simulink model "two_phase_main_loop"  (R2025b)
settings: Solver=daessc  StartTime=0  StopTime=50000
undefined symbols (not defined in the file): cfg, u_cmd
libraries: fl_lib x38, nesl_utility x26, SimscapeFluids_lib x11, slpidlib x2
(part 2 of 2)

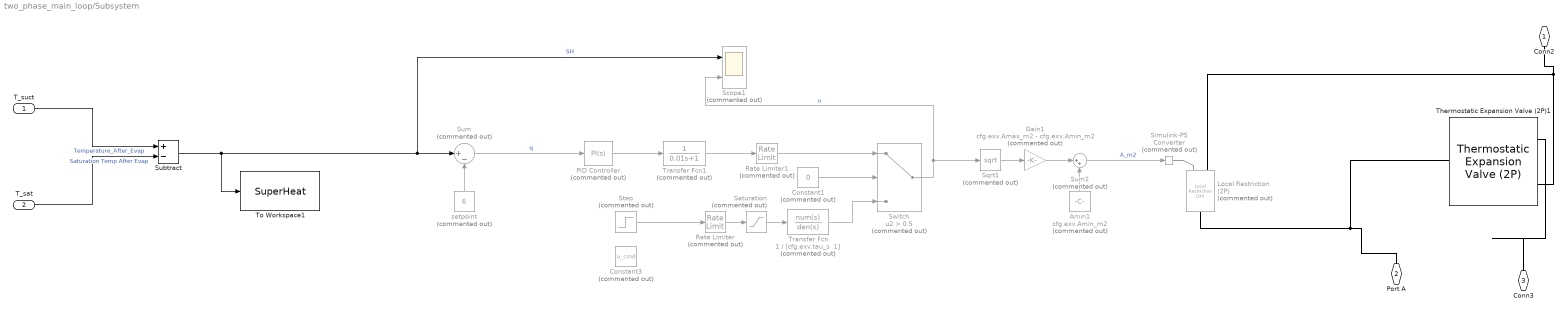
== system two_phase_main_loop/Subsystem ==
  T_suct : Inport
  T_sat : Inport  Port=2
  Amin1 : Constant  Commented=on  Value=cfg.exv.Amin_m2
  Constant1 : Constant  Commented=on  Value=0
  Constant3 : Constant  Commented=on  Value=u_cmd
  Gain1 : Gain  Commented=on  Gain=cfg.exv.Amax_m2 - cfg.exv.Amin_m2
  Local Restriction (2P) : fl_lib/Two-Phase Fluid/Elements/Local Restriction (2P)  Commented=on  restriction_type=foundation.enum.restriction_type.variable  restriction_area=1e-3 m^2  min_area="cfg.exv.Amin_m2  m^2"  max_area="cfg.exv.Amax_m2  m^2"  pressure_loss_model=foundation.enum.RestrictionPressureLossModel.Bernoulli  area=pi*0.02^2/4 m^2  Cd=0.64  B_lam=0.999
      settings: InternalSimscapePortConfiguration="{\"Bottom\":[],\"Left\":[{\"id\":\"A\",\"label\":\"A\",\"type\":\"foundation.two_phase_fluid.two_phase_fluid\"},{\"id\":\"area_in\",\"label\":\"AR\",\"type\":\"input\"}],\"Right\":[{\"id\":\"B\",\"label\":\"B\",\"type\":\"foundation.two_phase_fluid.two_phase_fluid\"}],\"Top\":[]}"
  PID Controller : slpidlib/PID Controller  Commented=on  Controller=PI  Form=Parallel  TimeDomain=Continuous-time  UseExternalTs=off  SampleTime=-1  IntegratorMethod=Forward Euler  FilterMethod=Forward Euler  ControllerParametersSource=internal  P=-0.05  I=- 0.001  UseKiTs=off  D=0  UseExternalDerivativeSource=off  N=100  UseFilter=on  TunerSelectOption=Transfer Function Based (PID Tuner App)  InitialConditionSource=internal  InitialConditionForIntegrator=0  InitialConditionForFilter=0  DifferentiatorICPrevScaledInput=0  ExternalReset=none  TrackingMode=off  Kt=1  LimitOutput=on  SatLimitsSource=internal  UpperSaturationLimit=1  LowerSaturationLimit=0  LinearizeAsGain=on  AntiWindupMode=clamping  Kb=1  LimitIntegrator=on  UpperIntegratorSaturationLimit=1  LowerIntegratorSaturationLimit=0  POutMin=[]  POutMax=[]  IOutMin=[]  IOutMax=[]  DOutMin=[]  DOutMax=[]  NOutMin=[]  NOutMax=[]  SumOutMin=[]  SumOutMax=[]  SaturationOutMin=[]  SaturationOutMax=[]  PParamMin=[]  PParamMax=[]  IParamMin=[]  IParamMax=[]  DParamMin=[]  DParamMax=[]  NParamMin=[]  NParamMax=[]  KbParamMin=[]  KbParamMax=[]  KtParamMin=[]  KtParamMax=[]  KbOutMin=[]  KbOutMax=[]  KtOutMin=[]  KtOutMax=[]  IntegratorOutMin=[]  IntegratorOutMax=[]  FilterOutMin=[]  FilterOutMax=[]  SumI1OutMin=[]  SumI1OutMax=[]  SumI2OutMin=[]  SumI2OutMax=[]  SumI3OutMin=[]  SumI3OutMax=[]  SumI4OutMin=[]  SumI4OutMax=[]  SumDOutMin=[]  SumDOutMax=[]  DifferentiatorOutMin=[]  DifferentiatorOutMax=[]  FilterDiffOutCoefMin=[]  FilterDiffOutCoefMax=[]  ReciprocalOutMin=[]  ReciprocalOutMax=[]  SumDenOutMin=[]  SumDenOutMax=[]  SumNumOutMin=[]  SumNumOutMax=[]  DivideOutMin=[]  DivideOutMax=[]  UdiffTsProdOutMin=[]  UdiffTsProdOutMax=[]  NTsProdOutMin=[]  NTsProdOutMax=[]  UintegralTsProdOutMin=[]  UintegralTsProdOutMax=[]  UngainTsProdOutMin=[]  UngainTsProdOutMax=[]  ClampingZeroOutDataTypeStr=Inherit: Inherit via back propagation  ClampingZeroOutMin=[]  ClampingZeroOutMax=[]  FilterDenConstantOutDataTypeStr=Inherit: Inherit via back propagation  FilterDenConstantOutMin=[]  FilterDenConstantOutMax=[]  PCopyOutDataTypeStr=Inherit: Inherit via back propagation  PCopyOutMin=[]  PCopyOutMax=[]  NCopyOutDataTypeStr=Inherit: Inherit via back propagation  NCopyOutMin=[]  NCopyOutMax=[]  IntegratorContinuousStateAttributes=''  IntegratorStateMustResolveToSignalObject=off  IntegratorRTWStateStorageClass=Auto  FilterContinuousStateAttributes=''  FilterStateMustResolveToSignalObject=off  FilterRTWStateStorageClass=Auto  ParallelPVariant=InternalParameters  IdealPVariant=Disabled  IVariant=InternalParameters  DVariant=Disabled  IntegratorVariant=Continuous  SatVariant=Enabled  AWVariant=ContClampingParallel  PCopyVariant=Disabled  TRVariant=Disabled  FdbkBlocksVariant=Forward  IdealPFdbkVariant=Disabled  SatFdbkVariant=Disabled  DerivativeFilterVariant=Disabled  NVariant=Disabled  NCopyVariant=Disabled_SignalSpec  FilterICVariant=Disabled  IntegratorICVariant=InternalICs  ExternalResetVariant=Disabled  TRSumVariant=Passthrough  SumFdbkVariant=Disabled  SumVariant=Sum_PI  TsampFilterVariant=InternalTs  TsampNgainVariant=Passthrough  TsampIntegralVariant=Disabled_SignalSpec  ExternalSaturationOutDataTypeStr=Inherit: Same as second input  DerivativeSourceVariant=Disabled  PreIntVariant=InternalPreInt
  Rate Limiter : RateLimiter  Commented=on  RisingSlewLimit=0.001  FallingSlewLimit=-0.001  SampleTimeMode=inherited  LinearizeAsGain=off
  Rate Limiter1 : RateLimiter  Commented=on  RisingSlewLimit=100  FallingSlewLimit=- 100  SampleTimeMode=inherited  LinearizeAsGain=off
  Saturation : Saturate  Commented=on  UpperLimit=cfg.exv.u_max  LowerLimit=0
  Scope1 : Scope  Commented=on  NumInputPorts=2
      settings: ActiveDisplayYMinimum=-231.24035158922058  ActiveDisplayYMaximum=311.50161349127353  DataLoggingVariableName=ScopeData3
  Simulink-PS Converter : nesl_utility/Simulink-PS Converter  Commented=on  PhysicalDomain=network_engine_domain  SubClassName=ps_input  LeftPortType=input  RightPortType=output  PseudoPeriodic=off  Frequencies=[]  NoiseDistribution=none  NoiseParameters=[]  Unit=m^2  AffineConversion=off  FilteringAndDerivatives=provide  SimscapeFilterOrder=1  InputFilterTimeConstant=0.001  UdotUserProvided=0
  Sqrt1 : Sqrt  Commented=on
  Step : Step  Commented=on  Time=600  Before=0.004  After=0.015  SampleTime=0
  Subtract : Sum  Inputs=+-
  Sum : Sum  Commented=on  Inputs=|+-
  Sum2 : Sum  Commented=on  Inputs=|++
  Switch : Switch  Commented=on  Criteria=u2 > Threshold  Threshold=0.5  SaturateOnIntegerOverflow=off  InputSameDT=off
  Thermostatic Expansion Valve (2P)1 : SimscapeFluids_lib/Two-Phase Fluid/Valves & Orifices/Flow Control Valves/Thermostatic Expansion Valve (2P)  valve_parameterization=fluids.two_phase_fluid.valves_orifices.flow_control_valves.enum.ThermostaticExpansionValveParameterization.Nominal  capacity_spec=fluids.two_phase_fluid.valves_orifices.flow_control_valves.enum.ThermostaticExpansionValveCapacitySpec.MassFlowRate  Q_nominal=63 kW  Q_max=70 kW  mdot_nominal=0.266 kg/s  mdot_max=0.4 kg/s  pressure_spec=fluids.two_phase_fluid.valves_orifices.flow_control_valves.enum.ThermostaticExpansionValvePressureSpec.SaturationTemperature  p_cond_nominal=1.5 MPa  p_evap_nominal=0.5 MPa  T_cond_nominal=55 degC  T_evap_nominal=5 degC  delta_T_sub=4 deltaK  delta_T_nominal=7 deltaK  delta_T_static=5 deltaK  mop=fluids.two_phase_fluid.valves_orifices.flow_control_valves.enum.ThermostaticExpansionValveMOP.Off  p_mop=0.5 MPa  T_mop=288.15 K  T_evap_out_TLU1=0 : 10 : 40 degC  p_bulb_TLU1=0.3 : 0.1 : 0.7 MPa  lift_TLU2=0 : 0.15 : 0.6 mm  p_evap_TLU2=0.3 : -0.05 : 0.1 MPa  lift_TLU3=0 : 0.15 : 0.6 mm  mdot_TLU3=0 : 0.015 : 0.06 kg/s  p_cond_ref=2 MPa  p_evap_ref=0.2 MPa  T_evap_out_ref=0 degC  delta_T_sub_ref=5 deltaK  pressure_equalization=fluids.two_phase_fluid.valves_orifices.flow_control_valves.enum.ThermostaticExpansionValveEqualization.Internal  bulb_dynamics=false  tau_bulb=20 s  leakage_fraction=1e-6  smoothing_factor=0.01  B_lam=0.999  tau_x=0.1 s  area=pi*0.02^2/4 m^2
      settings: InternalSimscapePortConfiguration="{\"Bottom\":[],\"Left\":[{\"id\":\"A\",\"label\":\"A\",\"type\":\"foundation.two_phase_fluid.two_phase_fluid\"}],\"Right\":[{\"id\":\"B\",\"label\":\"B\",\"type\":\"foundation.two_phase_fluid.two_phase_fluid\"}],\"Top\":[{\"id\":\"S\",\"label\":\"S\",\"type\":\"foundation.two_phase_fluid.two_phase_fluid\"}]}"
  To Workspace1 : ToWorkspace  VariableName=SuperHeat  SampleTime=-1
  Transfer Fcn : TransferFcn  Commented=on  Numerator=1  Denominator="[cfg.exv.tau_s  1]"
  Transfer Fcn1 : TransferFcn  Commented=on  Numerator=1  Denominator="[0.01  1]"
  setpoint : Constant  Commented=on  Value=6
  Conn2 : PMIOPort  Side=Left
  Port A : PMIOPort  Port=2  Side=Right
  Conn3 : PMIOPort  Port=3  Side=Right
  wires:
  Transfer Fcn1/1 -> Rate Limiter1/1
  Constant1/1 -> Switch/2
  Rate Limiter/1 -> Saturation/1
  Transfer Fcn/1 -> Switch/3
  Subtract/1 -> To Workspace1/1, Scope1/1, Sum/1  "SH"
  T_suct/1 -> Subtract/1  "Temperature_After_Evap"
  T_sat/1 -> Subtract/2  "Saturation Temp After Evap"
  setpoint/1 -> Sum/2
  Rate Limiter1/1 -> Switch/1
  Saturation/1 -> Transfer Fcn/1
  Sum/1 -> PID Controller/1  "q"
  PID Controller/1 -> Transfer Fcn1/1
  Switch/1 -> Sqrt1/1, Scope1/2  "u"
  Amin1/1 -> Sum2/2
  Gain1/1 -> Sum2/1
  Sum2/1 -> Simulink-PS Converter/1  "A_m2"
  Sqrt1/1 -> Gain1/1
  Step/1 -> Rate Limiter/1
  connections:
  Simulink-PS Converter/RConn1 -- Local Restriction (2P)/LConn2
  Conn3/RConn1 -- Thermostatic Expansion Valve (2P)1/LConn2
  Conn2/RConn1 -- Thermostatic Expansion Valve (2P)1/LConn1 -- Local Restriction (2P)/LConn1
  Port A/RConn1 -- Thermostatic Expansion Valve (2P)1/RConn1 -- Local Restriction (2P)/RConn1

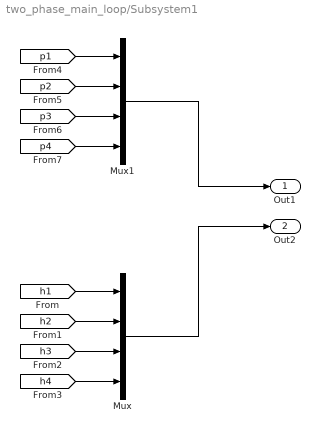
== system two_phase_main_loop/Subsystem1 ==
  Mux : Mux
  Mux1 : Mux
  Out1 : Outport
  Out2 : Outport  Port=2
  wires:
  [h1] -> Mux/1
  [p4] -> Mux1/4
  [p1] -> Mux1/1
  [h2] -> Mux/2
  [p3] -> Mux1/3
  [h4] -> Mux/4
  [p2] -> Mux1/2
  [h3] -> Mux/3
  Mux1/1 -> Out1/1
  Mux/1 -> Out2/1

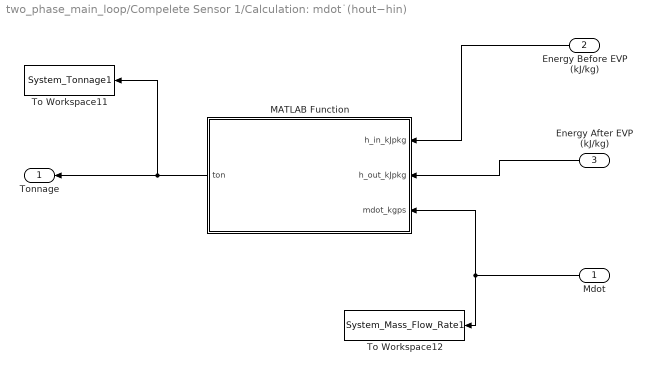
== system two_phase_main_loop/Compelete Sensor 1/Calculation: mdot˙(hout​−hin​) ==
  Mdot : Inport
  Energy Before EVP (kJ/kg) : Inport  Port=2
  "Energy After EVP (kJ/kg) " : Inport  Port=3
  MATLAB Function : MATLAB Function  TreatAsAtomicUnit=on
  To Workspace11 : ToWorkspace  VariableName=System_Tonnage1  SampleTime=-1
  To Workspace12 : ToWorkspace  VariableName=System_Mass_Flow_Rate1  SampleTime=-1
  Tonnage : Outport
  wires:
  MATLAB Function/1(ton) -> To Workspace11/1, Tonnage/1
  Mdot/1 -> To Workspace12/1, MATLAB Function/3(mdot_kgps)
  Energy Before EVP (kJ/kg)/1 -> MATLAB Function/1(h_in_kJpkg)
  "Energy After EVP (kJ/kg) "/1 -> MATLAB Function/2(h_out_kJpkg)

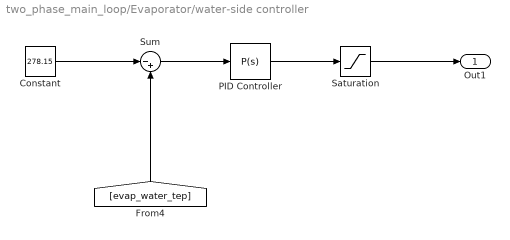
== system two_phase_main_loop/Evaporator/water-side controller ==
  Constant : Constant  Value=278.15
  PID Controller : slpidlib/PID Controller  Controller=P  Form=Parallel  TimeDomain=Continuous-time  UseExternalTs=off  SampleTime=-1  IntegratorMethod=Forward Euler  FilterMethod=Forward Euler  ControllerParametersSource=internal  P=0.005  I=1  UseKiTs=off  D=0  UseExternalDerivativeSource=off  N=100  UseFilter=on  TunerSelectOption=Transfer Function Based (PID Tuner App)  InitialConditionSource=internal  InitialConditionForIntegrator=0  InitialConditionForFilter=0  DifferentiatorICPrevScaledInput=0  ExternalReset=none  TrackingMode=off  Kt=1  LimitOutput=off  SatLimitsSource=internal  UpperSaturationLimit=inf  LowerSaturationLimit=-inf  LinearizeAsGain=on  AntiWindupMode=none  Kb=1  LimitIntegrator=off  UpperIntegratorSaturationLimit=inf  LowerIntegratorSaturationLimit=-inf  POutMin=[]  POutMax=[]  IOutMin=[]  IOutMax=[]  DOutMin=[]  DOutMax=[]  NOutMin=[]  NOutMax=[]  SumOutMin=[]  SumOutMax=[]  SaturationOutMin=[]  SaturationOutMax=[]  PParamMin=[]  PParamMax=[]  IParamMin=[]  IParamMax=[]  DParamMin=[]  DParamMax=[]  NParamMin=[]  NParamMax=[]  KbParamMin=[]  KbParamMax=[]  KtParamMin=[]  KtParamMax=[]  KbOutMin=[]  KbOutMax=[]  KtOutMin=[]  KtOutMax=[]  IntegratorOutMin=[]  IntegratorOutMax=[]  FilterOutMin=[]  FilterOutMax=[]  SumI1OutMin=[]  SumI1OutMax=[]  SumI2OutMin=[]  SumI2OutMax=[]  SumI3OutMin=[]  SumI3OutMax=[]  SumI4OutMin=[]  SumI4OutMax=[]  SumDOutMin=[]  SumDOutMax=[]  DifferentiatorOutMin=[]  DifferentiatorOutMax=[]  FilterDiffOutCoefMin=[]  FilterDiffOutCoefMax=[]  ReciprocalOutMin=[]  ReciprocalOutMax=[]  SumDenOutMin=[]  SumDenOutMax=[]  SumNumOutMin=[]  SumNumOutMax=[]  DivideOutMin=[]  DivideOutMax=[]  UdiffTsProdOutMin=[]  UdiffTsProdOutMax=[]  NTsProdOutMin=[]  NTsProdOutMax=[]  UintegralTsProdOutMin=[]  UintegralTsProdOutMax=[]  UngainTsProdOutMin=[]  UngainTsProdOutMax=[]  ClampingZeroOutDataTypeStr=Inherit: Inherit via back propagation  ClampingZeroOutMin=[]  ClampingZeroOutMax=[]  FilterDenConstantOutDataTypeStr=Inherit: Inherit via back propagation  FilterDenConstantOutMin=[]  FilterDenConstantOutMax=[]  PCopyOutDataTypeStr=Inherit: Inherit via back propagation  PCopyOutMin=[]  PCopyOutMax=[]  NCopyOutDataTypeStr=Inherit: Inherit via back propagation  NCopyOutMin=[]  NCopyOutMax=[]  IntegratorContinuousStateAttributes=''  IntegratorStateMustResolveToSignalObject=off  IntegratorRTWStateStorageClass=Auto  FilterContinuousStateAttributes=''  FilterStateMustResolveToSignalObject=off  FilterRTWStateStorageClass=Auto  ParallelPVariant=InternalParameters  IdealPVariant=Disabled  IVariant=Disabled  DVariant=Disabled  IntegratorVariant=Disabled  SatVariant=Disabled  AWVariant=Disabled  PCopyVariant=Disabled  TRVariant=Disabled  FdbkBlocksVariant=Forward  IdealPFdbkVariant=Disabled  SatFdbkVariant=Disabled  DerivativeFilterVariant=Disabled  NVariant=Disabled  NCopyVariant=Disabled_SignalSpec  FilterICVariant=Disabled  IntegratorICVariant=Disabled  ExternalResetVariant=Disabled  TRSumVariant=Passthrough  SumFdbkVariant=Disabled  SumVariant=Passthrough_P  TsampFilterVariant=InternalTs  TsampNgainVariant=Passthrough  TsampIntegralVariant=Disabled_SignalSpec  ExternalSaturationOutDataTypeStr=Inherit: Same as second input  DerivativeSourceVariant=Disabled  PreIntVariant=InternalPreInt
  Saturation : Saturate  UpperLimit=2.7  LowerLimit=0.09
  Sum : Sum  Inputs=|-+
  Out1 : Outport
  wires:
  Saturation/1 -> Out1/1
  Constant/1 -> Sum/1
  [evap_water_tep] -> Sum/2
  Sum/1 -> PID Controller/1
  PID Controller/1 -> Saturation/1

== matlab function two_phase_main_loop/Compelete Sensor 1/Calculation: mdot˙(hout​−hin​)/MATLAB Function ==
  data: h_in_kJpkg input; ton output; h_out_kJpkg input; mdot_kgps input
function ton = calc_tonnage(h_in_kJpkg, h_out_kJpkg, mdot_kgps)
%   calc_tonnage  Computes system capacity in refrigeration tons.
%
%   ton = calc_tonnage(h_in_kJpkg, h_out_kJpkg, mdot_kgps, mode)
%
%   Inputs
%   -------
%   h_in_kJpkg   : inlet specific enthalpy  [kJ/kg]
%   h_out_kJpkg  : outlet specific enthalpy [kJ/kg]
%   mdot_kgps    : mass flow rate           [kg/s]
%
%   Output
%   -------
%   ton          : capacity in refrigeration tons [TR]
%
%   Notes
%   -----
%   • For evaporators (cooling): Q̇ = ṁ × (h_out − h_in)
%   • 1 ton refrigeration = 3.517 kW
%
%   Example
%   -------
%       ton_cool = calc_tonnage(250, 430, 0.05);
%


Qdot_kW = mdot_kgps .* (h_out_kJpkg - h_in_kJpkg); % kJ/kg × kg/s = kJ/s = kW


ton = Qdot_kW ./ 3.517; % Convert to refrigeration tons

end
